simulink model "Simulink_2021b"  (R2023b)
settings: Solver=ode23s  StartTime=0.0  StopTime=10.0  RelTol=1e-3
libraries: simulink x1
settings Model: Creator=tweingar  LastModifiedBy=looki
settings SolverCC: AlgebraicLoopSolver=TrustRegion
settings DebuggingCC: UnconnectedInputMsg=warning  UnconnectedOutputMsg=warning  UnconnectedLineMsg=warning
settings ModelReferenceCC: EnableRefExpFcnMdlSchedulingChecks=on
settings RTWCC: DLArmComputeVersion=19.05

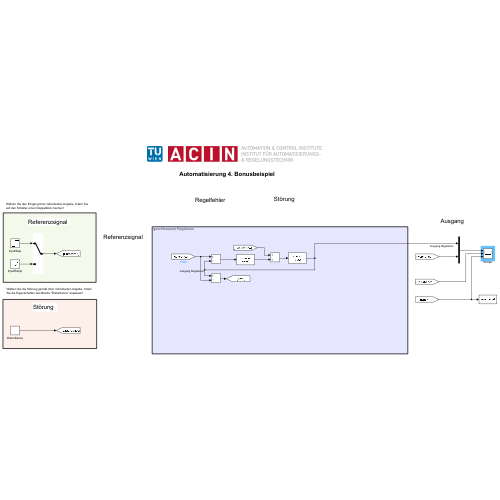
[thumbnail: Simulink's stored preview of the top-level diagram]
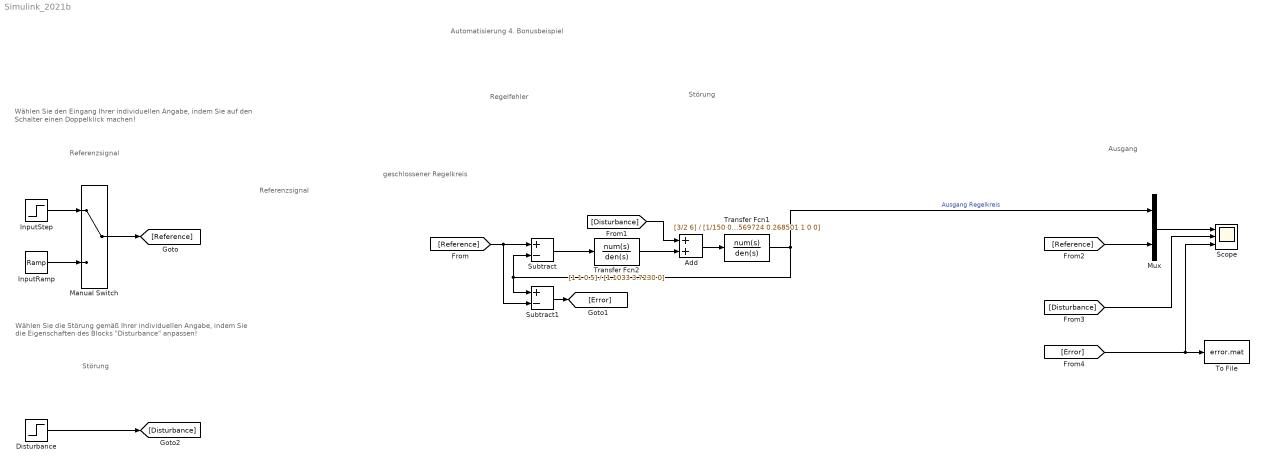
== system Simulink_2021b ==
  note: Wählen Sie den Eingang Ihrer individuellen Angabe, indem Sie auf den Schalter einen Doppelklick machen!
  note: geschlossener Regelkreis
  note: Störung
  note: Referenzsignal
  note: Ausgang
  note: Störung
  note: Automatisierung 4. Bonusbeispiel
  note: Regelfehler
  note: Wählen Sie die Störung gemäß Ihrer individuellen Angabe, indem Sie die Eigenschaften des Blocks "Disturbance" anpassen!
  note: Referenzsignal
  Add : Sum
  Disturbance : Step  Time=5  After=0.01  SampleTime=0
  InputRamp : simulink/Sources/Ramp  slope=1  start=1  InitialOutput=0
  InputStep : Step  SampleTime=0
  Manual Switch : ManualSwitch
  Mux : Mux  Inputs=2
  Scope : Scope  NumInputPorts=3
  Subtract : Sum  Inputs=+-
  Subtract1 : Sum  Inputs=+-
  To File : ToFile  Filename=error.mat  MatrixName=error  SaveFormat=Timeseries
  Transfer Fcn1 : TransferFcn  Numerator=[3/2 6]  Denominator=[1/150 0.0569724 0.268501 1 0 0]
  Transfer Fcn2 : TransferFcn  Numerator=[1 1 0.5]  Denominator=[1.1033 3.7230 0]
  wires:
  Disturbance/1 -> [Disturbance]
  Mux/1 -> Scope/1
  InputStep/1 -> Manual Switch/1
  InputRamp/1 -> Manual Switch/2
  Manual Switch/1 -> [Reference]
  [Reference] -> Mux/2
  [Disturbance] -> Scope/2
  [Error] -> To File/1, Scope/3
  Subtract1/1 -> [Error]
  Subtract/1 -> Transfer Fcn2/1
  [Disturbance] -> Add/1
  Transfer Fcn1/1 -> Mux/1, Subtract1/1, Subtract/2  "Ausgang Regelkreis"
  [Reference] -> Subtract/1, Subtract1/2
  Add/1 -> Transfer Fcn1/1
  Transfer Fcn2/1 -> Add/2
